simulink model "ROBOT3EJES"  (R2025a)
settings: Solver=VariableStepAuto  StartTime=0.0  StopTime=3  RelTol=1e-3
model workspace: external: MATLAB File C:\Users\ernes\Desktop\CUCEI\4TO\Seminario modelado y Simulacion\PROYECTO MOD.SIM\ROBOT3EJES_DataFile.m (data not in the file)
undefined symbols (not defined in the file): smiData, X, Y, Z
libraries: fl_lib x40, nesl_utility x28, sm_lib x20, ee_lib x13
(part 2 of 2)

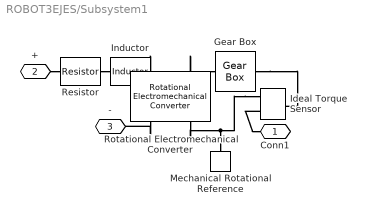
== system ROBOT3EJES/Subsystem1 ==
  Gear Box : fl_lib/Mechanical/Mechanisms/Gear Box  ratio=150  t_in_specify=off  t_in_priority=None  t_in=0 N*m  t_in_nominal_specify=off  t_in_nominal_value=1  t_in_nominal_unit=N*m  t_out_specify=off  t_out_priority=None  t_out=0 N*m  t_out_nominal_specify=off  t_out_nominal_value=1  t_out_nominal_unit=N*m
  Ideal Torque Sensor : fl_lib/Mechanical/Mechanical Sensors/Ideal Torque Sensor
  Inductor : fl_lib/Electrical/Electrical Elements/Inductor  l=23 mH  r=0 Ohm  g=1e-9 1/Ohm  i_specify=off  i_priority=None  i=0 A  i_nominal_specify=off  i_nominal_value=1  i_nominal_unit=A  v_specify=off  v_priority=None  v=0 V  v_nominal_specify=off  v_nominal_value=1  v_nominal_unit=V  i_L_specify=off  i_L_priority=High  i_L=0 A  i_L_nominal_specify=off  i_L_nominal_value=1  i_L_nominal_unit=A
  Mechanical Rotational Reference : fl_lib/Mechanical/Rotational Elements/Mechanical Rotational Reference
  Resistor : fl_lib/Electrical/Electrical Elements/Resistor  R=2 Ohm  i_specify=off  i_priority=None  i=0 A  i_nominal_specify=off  i_nominal_value=1  i_nominal_unit=A  v_specify=off  v_priority=None  v=0 V  v_nominal_specify=off  v_nominal_value=1  v_nominal_unit=V
  Rotational Electromechanical Converter : fl_lib/Electrical/Electrical Elements/Rotational Electromechanical Converter  K=1 V*s/rad  i_specify=off  i_priority=None  i=0 A  i_nominal_specify=off  i_nominal_value=1  i_nominal_unit=A  v_specify=off  v_priority=None  v=0 V  v_nominal_specify=off  v_nominal_value=1  v_nominal_unit=V  t_specify=off  t_priority=None  t=0 N*m  t_nominal_specify=off  t_nominal_value=1  t_nominal_unit=N*m  w_specify=off  w_priority=None  w=0 rad/s  w_nominal_specify=off  w_nominal_value=1  w_nominal_unit=rad/s
  Conn1 : PMIOPort  Side=Right
  + : PMIOPort  Port=2  Side=Left
  - : PMIOPort  Port=3  Side=Left
  connections:
  Ideal Torque Sensor/RConn2 -- Conn1/RConn1
  Rotational Electromechanical Converter/LConn1 -- Inductor/RConn1
  Rotational Electromechanical Converter/RConn1 -- -/RConn1
  Ideal Torque Sensor/RConn1 -- Rotational Electromechanical Converter/RConn2 -- Mechanical Rotational Reference/LConn1
  Resistor/RConn1 -- Inductor/LConn1
  +/RConn1 -- Resistor/LConn1
  Rotational Electromechanical Converter/LConn2 -- Gear Box/LConn1
  Gear Box/RConn1 -- Ideal Torque Sensor/LConn1

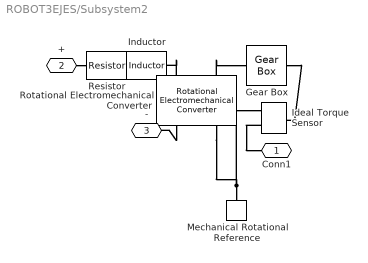
== system ROBOT3EJES/Subsystem2 ==
  Gear Box : fl_lib/Mechanical/Mechanisms/Gear Box  ratio=150  t_in_specify=off  t_in_priority=None  t_in=0 N*m  t_in_nominal_specify=off  t_in_nominal_value=1  t_in_nominal_unit=N*m  t_out_specify=off  t_out_priority=None  t_out=0 N*m  t_out_nominal_specify=off  t_out_nominal_value=1  t_out_nominal_unit=N*m
  Ideal Torque Sensor : fl_lib/Mechanical/Mechanical Sensors/Ideal Torque Sensor
  Inductor : fl_lib/Electrical/Electrical Elements/Inductor  l=23 mH  r=0 Ohm  g=1e-9 1/Ohm  i_specify=off  i_priority=None  i=0 A  i_nominal_specify=off  i_nominal_value=1  i_nominal_unit=A  v_specify=off  v_priority=None  v=0 V  v_nominal_specify=off  v_nominal_value=1  v_nominal_unit=V  i_L_specify=off  i_L_priority=High  i_L=0 A  i_L_nominal_specify=off  i_L_nominal_value=1  i_L_nominal_unit=A
  Mechanical Rotational Reference : fl_lib/Mechanical/Rotational Elements/Mechanical Rotational Reference
  Resistor : fl_lib/Electrical/Electrical Elements/Resistor  R=2 Ohm  i_specify=off  i_priority=None  i=0 A  i_nominal_specify=off  i_nominal_value=1  i_nominal_unit=A  v_specify=off  v_priority=None  v=0 V  v_nominal_specify=off  v_nominal_value=1  v_nominal_unit=V
  Rotational Electromechanical Converter : fl_lib/Electrical/Electrical Elements/Rotational Electromechanical Converter  K=1 V*s/rad  i_specify=off  i_priority=None  i=0 A  i_nominal_specify=off  i_nominal_value=1  i_nominal_unit=A  v_specify=off  v_priority=None  v=0 V  v_nominal_specify=off  v_nominal_value=1  v_nominal_unit=V  t_specify=off  t_priority=None  t=0 N*m  t_nominal_specify=off  t_nominal_value=1  t_nominal_unit=N*m  w_specify=off  w_priority=None  w=0 rad/s  w_nominal_specify=off  w_nominal_value=1  w_nominal_unit=rad/s
  Conn1 : PMIOPort  Side=Right
  + : PMIOPort  Port=2  Side=Left
  - : PMIOPort  Port=3  Side=Left
  connections:
  Ideal Torque Sensor/RConn2 -- Conn1/RConn1
  Rotational Electromechanical Converter/LConn1 -- Inductor/RConn1
  Rotational Electromechanical Converter/RConn1 -- -/RConn1
  Mechanical Rotational Reference/LConn1 -- Ideal Torque Sensor/RConn1 -- Rotational Electromechanical Converter/RConn2
  Resistor/RConn1 -- Inductor/LConn1
  +/RConn1 -- Resistor/LConn1
  Rotational Electromechanical Converter/LConn2 -- Gear Box/LConn1
  Gear Box/RConn1 -- Ideal Torque Sensor/LConn1
